simulink model "exercicio3"  (R2015a)
settings: Solver=ode45  StartTime=0.0  StopTime=10000.0  RelTol=1e-3
libraries: commrandsrc2 x2, commsink2 x2, commdigbbndfm2 x2, commchan3 x1, commrflib2 x1
settings Model: Creator=francisco  LastModifiedBy=francisco

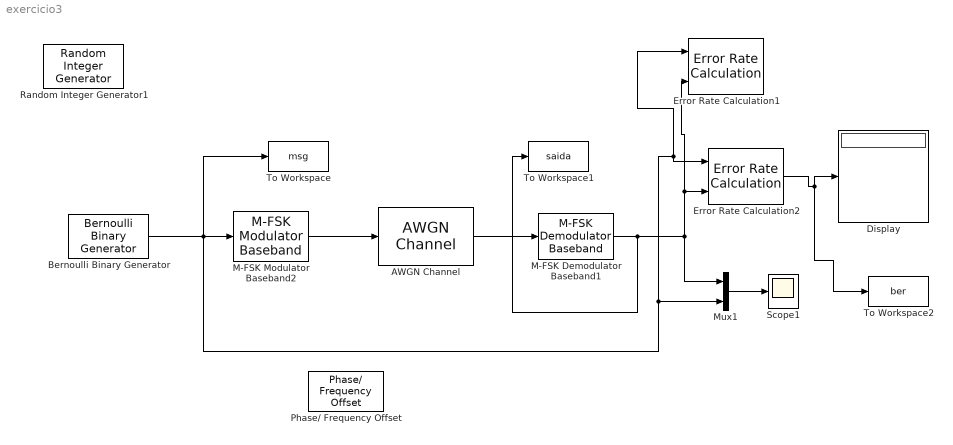
== system exercicio3 ==
  AWGN Channel : commchan3/AWGN Channel  InputProcessing=Columns as channels (frame based)  seed=67  noiseMode="Signal to noise ratio  (Eb/No)"  EbNodB=EbNo  EsNodB=10  SNRdB=10  bitsPerSym=5  Ps=1  Tsym=1  variance=1
  Bernoulli Binary Generator : commrandsrc2/Bernoulli Binary Generator  P=0.5  seed=61  Ts=1  frameBased=off  sampPerFrame=1  orient=off  outDataType=double
  Display : Display
  Error Rate Calculation1 : commsink2/Error Rate Calculation  N=0  st_delay=0  cp_mode=Entire frame  subframe=[]  PMode=Workspace  WsName=ErrorVec  RsMode2=off  stop=off  numErr=100  maxBits=1e6
  Error Rate Calculation2 : commsink2/Error Rate Calculation  N=0  st_delay=0  cp_mode=Entire frame  subframe=[]  PMode=Port  WsName=ErrorVec  RsMode2=off  stop=off  numErr=100  maxBits=1e6
  M-FSK Demodulator Baseband1 : commdigbbndfm2/M-FSK Demodulator Baseband  M=8  OutType=Integer  Dec=Gray  freqSep=6  numSamp=200  RateOptions=Enforce single-rate processing  outDataType=double
  M-FSK Modulator Baseband2 : commdigbbndfm2/M-FSK Modulator Baseband  M=8  InType=Integer  Enc=Gray  freqSep=6  phaseType=Continuous  numSamp=200  RateOptions=Enforce single-rate processing  outDataType=double
  Mux1 : Mux  Inputs=2
  Phase/ Frequency Offset : commrflib2/Phase// Frequency Offset  phaseOffset=10  freqPort=off  freqOffset=0
  Random Integer Generator1 : commrandsrc2/Random Integer Generator  RequirementInfo={} %GIDa_5080aef8_8719_4c24_ab1b_0732f3582dbc  mul=2  seed=37  Ts=1  frameBased=off  sampPerFrame=1  orient=off  outDataType=double
  Scope1 : Scope
      settings: SaveName=ScopeData2  Decimation=100
  To Workspace : ToWorkspace  VariableName=msg  SaveFormat=Timeseries  SampleTime=-1
  To Workspace1 : ToWorkspace  VariableName=saida  SaveFormat=Timeseries  SampleTime=-1
  To Workspace2 : ToWorkspace  VariableName=ber  SampleTime=-1
      settings: MaxDataPoints=2  Save2DSignal=2-D array (concatenate along first dimension)
  wires:
  Bernoulli Binary Generator/1 -> M-FSK Modulator Baseband2/1, To Workspace/1, Error Rate Calculation1/1, Error Rate Calculation2/1, Mux1/2
  M-FSK Demodulator Baseband1/1 -> To Workspace1/1, Error Rate Calculation1/2, Error Rate Calculation2/2, Mux1/1
  Mux1/1 -> Scope1/1
  Error Rate Calculation2/1 -> To Workspace2/1, Display/1
  AWGN Channel/1 -> M-FSK Demodulator Baseband1/1
  M-FSK Modulator Baseband2/1 -> AWGN Channel/1
